simulink model "ex4simc"  (R2015a)
settings: Solver=ode45  StartTime=0.0  StopTime=10.0  RelTol=1e-3
values from neighbouring files (symbols this model uses):
  A = [0, 1; 0, 0]    [ex4.m]
  B = [0; -m*g*d/(L*(J/R^2 + m))]    [ex4.m]
  C = K*(s+a)/s    [ex1.m]    (also in ex4.m = [1, 0])
  K = 2    [ex1.m]    (also in ex2.m = 0.522220481487; ex4.m = acker(sysd.A, sysd.B, poles))
settings Model: Creator=BPeixoto  LastModifiedBy=BPeixoto

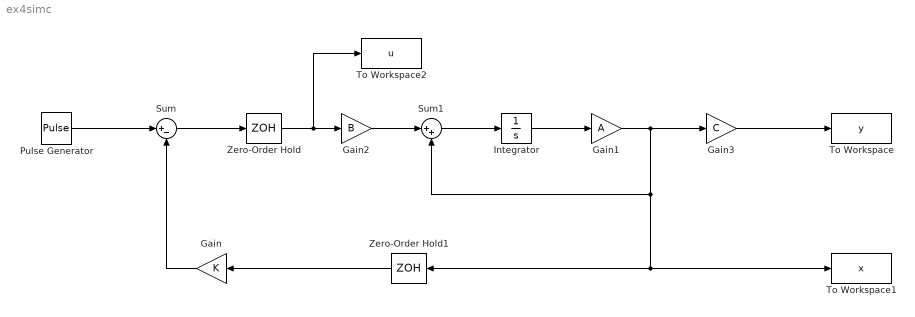
== system ex4simc ==
  Gain : Gain  Gain=K
  Gain1 : Gain  Gain=A
  Gain2 : Gain  Gain=B
  Gain3 : Gain  Gain=C
  Integrator : Integrator
  Pulse Generator : DiscretePulseGenerator  PulseType=Time based  Period=10  PulseWidth=5
  Sum : Sum  Inputs=|+-
  Sum1 : Sum  Inputs=|++
  To Workspace : ToWorkspace  VariableName=y  SaveFormat=Timeseries  SampleTime=-1
  To Workspace1 : ToWorkspace  VariableName=x  SaveFormat=Timeseries  SampleTime=-1
  To Workspace2 : ToWorkspace  VariableName=u  SaveFormat=Timeseries  SampleTime=-1
  Zero-Order Hold : ZeroOrderHold
  Zero-Order Hold1 : ZeroOrderHold
  wires:
  Pulse Generator/1 -> Sum/1
  Sum/1 -> Zero-Order Hold/1
  Gain/1 -> Sum/2
  Integrator/1 -> Gain1/1
  Sum1/1 -> Integrator/1
  Zero-Order Hold/1 -> To Workspace2/1, Gain2/1
  Gain2/1 -> Sum1/1
  Gain3/1 -> To Workspace/1
  Gain1/1 -> Gain3/1, Zero-Order Hold1/1, To Workspace1/1, Sum1/2
  Zero-Order Hold1/1 -> Gain/1
